simulink model "gm_Dynamic_Calculations"  (R2018a)
settings: Solver=ode3  StartTime=0.0  StopTime=0.06  RelTol=1e-3  EnableMultiTasking=on
libraries: hdlsllib x4, hdlmdlgenlib x4, simulink x1
settings Model: Creator=Estra  LastModifiedBy=Talha Rao
settings SolverCC: PositivePriorityOrder=on
settings DataIOCC: LimitDataPoints=on  SaveFormat=Array  SaveOutput=off  SaveTime=off
settings OptimizationCC: BlockReduction=off  ConditionallyExecuteInputs=off  DefaultParameterBehavior=Inlined  UseDivisionForNetSlopeComputation=on  UseFloatMulNetSlope=on  InlineInvariantSignals=on  PassReuseOutputArgsAs=Individual arguments  ExpressionDepthLimit=2147483647  ZeroExternalMemoryAtStartup=off  ZeroInternalMemoryAtStartup=off  NoFixptDivByZeroProtection=on  EfficientFloat2IntCast=on  LifeSpan=1  MaxStackSize=64
settings DebuggingCC: SignalInfNanChecking=warning  UnderspecifiedInitializationDetection=Classic  MergeDetectMultiDrivingBlocksExec=none  SolverPrmCheckMsg=warning  InheritedTsInSrcMsg=none  ParameterTunabilityLossMsg=error  UniqueDataStoreMsg=warning  AllowSymbolicDim=off  StateNameClashWarn=warning  SFUnexpectedBacktrackingDiag=warning  SFNoUnconditionalDefaultTransitionDiag=warning  SFExecutionAtInitializationDiag=none
settings HardwareCC: ProdBitPerPointer=32  ProdBitPerSizeT=32  ProdBitPerPtrDiffT=32  ProdLargestAtomicInteger=Long  ProdLargestAtomicFloat=Double  ProdWordSize=32  ProdLongLongMode=on  ProdHWDeviceType=ARM Compatible->ARM Cortex  TargetBitPerPointer=64  TargetBitPerSizeT=64  TargetBitPerPtrDiffT=64  TargetLongLongMode=on  TargetIntDivRoundTo=Zero  TargetEndianess=LittleEndian  TargetWordSize=64  TargetHWDeviceType=Custom Processor->MATLAB Host Computer  ProdEqTarget=off
settings ModelReferenceCC: PropagateSignalLabelsOutOfModel=off
settings SFSimCC: MATLABDynamicMemAlloc=off
settings RTWCC: SystemTargetFile=ert.tlc  HardwareBoard=Xilinx Zynq-7000 based board  TLCOptions="-aInlineSetEventsForThisBaseRateFcn=TLC_FALSE -aSuppressMultiTaskScheduler=TLC_FALSE  -aRateBasedStepFcn=0"  TemplateMakefile=ert_default_tmf  GenerateReport=on  Toolchain=Xilinx Software Development Kit (SDK)  IncludeHyperlinkInReport=on  LaunchReport=on  GenerateTraceInfo=on  GenerateTraceReport=on  GenerateTraceReportSl=on  GenerateTraceReportSf=on  GenerateTraceReportEml=on  GenerateCodeMetricsReport=on
settings CodeAppCC: ForceParamTrailComments=on  IgnoreCustomStorageClasses=off  OperatorAnnotations=on  SimulinkDataObjDesc=on  SFDataObjDesc=on  CustomSymbolStrGlobalVar=rt$N$M  CustomSymbolStrType=$N$M  CustomSymbolStrFcn=$N$M$F  CustomSymbolStrMacro=$N$M  InsertBlockDesc=on
settings ERTTargetCC: IncludeMdlTerminateFcn=off  CombineSignalStateStructs=on  SupportAbsoluteTime=off  SupportComplex=off  SupportNonInlinedSFcns=on  SupportVariableSizeSignals=on  InlinedParameterPlacement=NonHierarchical  ERTFilePackagingFormat=CompactWithDataFile
settings ConfigComp: CovMetricSettings=dw  CovHtmlReporting=on  CovSaveCumulativeToWorkspaceVar=on  CovSaveSingleToWorkspaceVar=on  CovExternalEMLEnable=off

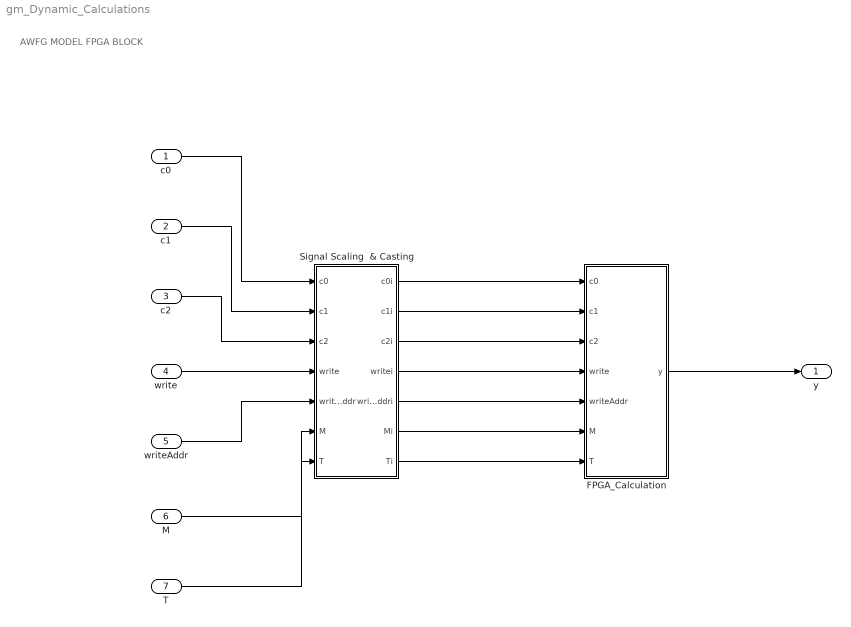
== system gm_Dynamic_Calculations ==
  note: AWFG MODEL FPGA BLOCK
  c0 : Inport  OutDataTypeStr=int32  PortDimensions=1  SampleTime=1e-08
  c1 : Inport  Port=2  OutDataTypeStr=int32  PortDimensions=1  SampleTime=1e-08
  c2 : Inport  Port=3  OutDataTypeStr=int32  PortDimensions=1  SampleTime=1e-08
  write : Inport  Port=4  OutDataTypeStr=boolean  PortDimensions=1  SampleTime=1e-08
  writeAddr : Inport  Port=5  OutDataTypeStr=uint8  PortDimensions=1  SampleTime=1e-08
  M : Inport  Port=6  OutDataTypeStr=int32  PortDimensions=1  SampleTime=1e-08
  T : Inport  Port=7  OutDataTypeStr=uint32  PortDimensions=1  SampleTime=1e-08
  FPGA_Calculation : Subsystem
  Signal Scaling  & Casting : Subsystem
  y : Outport  OutDataTypeStr=fixdt(1,27,19)  PortDimensions=[1 1]  SampleTime=[1e-08,0]
  wires:
  c0/1 -> Signal Scaling  & Casting/1(c0)
  c1/1 -> Signal Scaling  & Casting/2(c1)
  c2/1 -> Signal Scaling  & Casting/3(c2)
  write/1 -> Signal Scaling  & Casting/4(write)
  writeAddr/1 -> Signal Scaling  & Casting/5(writeAddr)
  M/1 -> Signal Scaling  & Casting/6(M)
  T/1 -> Signal Scaling  & Casting/7(T)
  FPGA_Calculation/1(y) -> y/1
  Signal Scaling  & Casting/1(c0i) -> FPGA_Calculation/1(c0)
  Signal Scaling  & Casting/2(c1i) -> FPGA_Calculation/2(c1)
  Signal Scaling  & Casting/3(c2i) -> FPGA_Calculation/3(c2)
  Signal Scaling  & Casting/4(writei) -> FPGA_Calculation/4(write)
  Signal Scaling  & Casting/5(writeAddri) -> FPGA_Calculation/5(writeAddr)
  Signal Scaling  & Casting/6(Mi) -> FPGA_Calculation/6(M)
  Signal Scaling  & Casting/7(Ti) -> FPGA_Calculation/7(T)

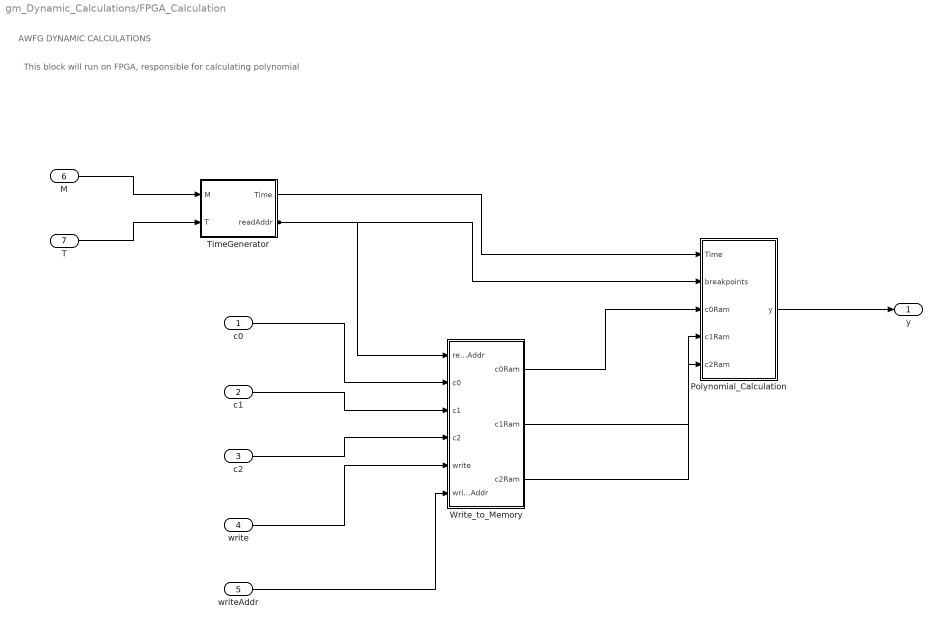
== system gm_Dynamic_Calculations/FPGA_Calculation ==
  note: AWFG DYNAMIC CALCULATIONS
  note: This block will run on FPGA, responsible for calculating polynomial
  c0 : Inport  PortDimensions=1  SampleTime=1e-08
  c1 : Inport  Port=2  PortDimensions=1  SampleTime=1e-08
  c2 : Inport  Port=3  PortDimensions=1  SampleTime=1e-08
  write : Inport  Port=4  PortDimensions=1  SampleTime=1e-08
  writeAddr : Inport  Port=5  PortDimensions=1  SampleTime=1e-08
  M : Inport  Port=6  PortDimensions=1  SampleTime=1e-08
  T : Inport  Port=7  PortDimensions=1  SampleTime=1e-08
  Polynomial_Calculation : Subsystem
  TimeGenerator : Subsystem
  Write_to_Memory : Subsystem
  y : Outport
  wires:
  c0/1 -> Write_to_Memory/2(c0)
  c1/1 -> Write_to_Memory/3(c1)
  c2/1 -> Write_to_Memory/4(c2)
  write/1 -> Write_to_Memory/5(write)
  writeAddr/1 -> Write_to_Memory/6(writeAddr)
  M/1 -> TimeGenerator/1(M)
  T/1 -> TimeGenerator/2(T)
  Polynomial_Calculation/1(y) -> y/1
  TimeGenerator/1(Time) -> Polynomial_Calculation/1(Time)
  TimeGenerator/2(readAddr) -> Polynomial_Calculation/2(breakpoints), Write_to_Memory/1(readAddr)
  Write_to_Memory/1(c0Ram) -> Polynomial_Calculation/3(c0Ram)
  Write_to_Memory/2(c1Ram) -> Polynomial_Calculation/4(c1Ram)
  Write_to_Memory/3(c2Ram) -> Polynomial_Calculation/5(c2Ram)

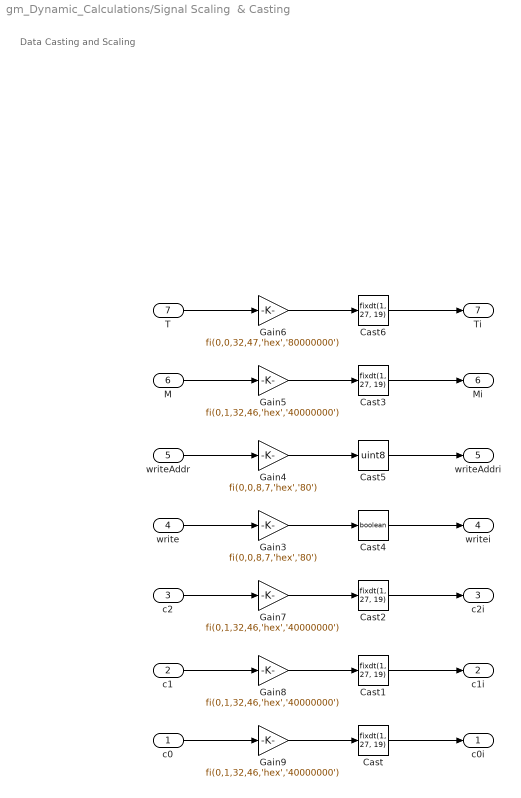
== system gm_Dynamic_Calculations/Signal Scaling  & Casting ==
  note: Data Casting and Scaling
  c0 : Inport  PortDimensions=1  SampleTime=1e-08
  c1 : Inport  Port=2  PortDimensions=1  SampleTime=1e-08
  c2 : Inport  Port=3  PortDimensions=1  SampleTime=1e-08
  write : Inport  Port=4  PortDimensions=1  SampleTime=1e-08
  writeAddr : Inport  Port=5  PortDimensions=1  SampleTime=1e-08
  M : Inport  Port=6  PortDimensions=1  SampleTime=1e-08
  T : Inport  Port=7  PortDimensions=1  SampleTime=1e-08
  Cast{,1..3,6} (5 alike) : DataTypeConversion  OutDataTypeStr=fixdt(1, 27, 19)  SampleTime=1e-08
  Cast4 : DataTypeConversion  OutDataTypeStr=boolean  SampleTime=1e-08
  Cast5 : DataTypeConversion  OutDataTypeStr=uint8  SampleTime=1e-08
  Gain3 : Gain  Gain=fi(0,0,8,7,'hex','80')  ParamDataTypeStr=fixdt(0, 8, 7)  OutDataTypeStr=fixdt(0, 8, 7)  SampleTime=1e-08
  Gain4 : Gain  Gain=fi(0,0,8,7,'hex','80')  ParamDataTypeStr=fixdt(0, 8, 7)  OutDataTypeStr=fixdt(0, 16, 7)  SampleTime=1e-08
  Gain{5,7..9} (4 alike) : Gain  Gain=fi(0,1,32,46,'hex','40000000')  ParamDataTypeStr=fixdt(1, 32, 46)  OutDataTypeStr=fixdt(1, 64, 46)  SampleTime=1e-08
  Gain6 : Gain  Gain=fi(0,0,32,47,'hex','80000000')  ParamDataTypeStr=fixdt(0, 32, 47)  OutDataTypeStr=fixdt(0, 64, 47)  SampleTime=1e-08
  c0i : Outport
  c1i : Outport  Port=2
  c2i : Outport  Port=3
  writei : Outport  Port=4
  writeAddri : Outport  Port=5
  Mi : Outport  Port=6
  Ti : Outport  Port=7
  wires:
  c0/1 -> Gain9/1
  c1/1 -> Gain8/1
  c2/1 -> Gain7/1
  write/1 -> Gain3/1
  writeAddr/1 -> Gain4/1
  M/1 -> Gain5/1
  T/1 -> Gain6/1
  Cast/1 -> c0i/1
  Cast1/1 -> c1i/1
  Cast2/1 -> c2i/1
  Cast3/1 -> Mi/1
  Cast4/1 -> writei/1
  Cast5/1 -> writeAddri/1
  Cast6/1 -> Ti/1
  Gain3/1 -> Cast4/1
  Gain4/1 -> Cast5/1
  Gain5/1 -> Cast3/1
  Gain6/1 -> Cast6/1
  Gain7/1 -> Cast2/1
  Gain8/1 -> Cast1/1
  Gain9/1 -> Cast/1

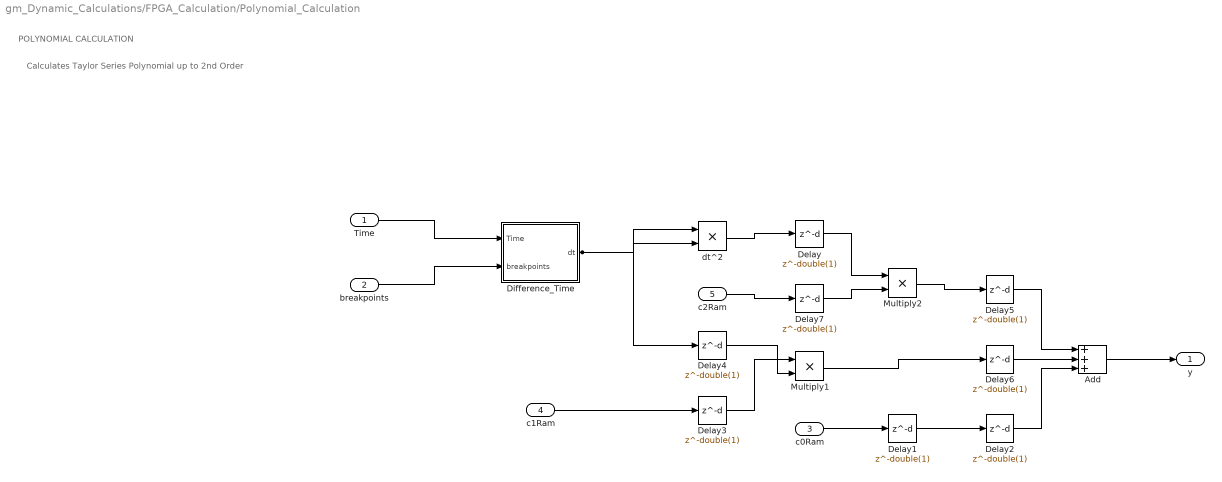
== system gm_Dynamic_Calculations/FPGA_Calculation/Polynomial_Calculation ==
  note: POLYNOMIAL CALCULATION
  note: Calculates Taylor Series Polynomial up to 2nd Order
  Time : Inport  PortDimensions=1  SampleTime=1e-08
  breakpoints : Inport  Port=2  PortDimensions=1  SampleTime=1e-08
  c0Ram : Inport  Port=3  PortDimensions=1  SampleTime=1e-08
  c1Ram : Inport  Port=4  PortDimensions=1  SampleTime=1e-08
  c2Ram : Inport  Port=5  PortDimensions=1  SampleTime=1e-08
  Add : Sum  Inputs=+++  AccumDataTypeStr=fixdt(1, 32, 19)  OutDataTypeStr=fixdt(1, 27, 19)  SampleTime=1e-08
  Delay{,1..7} (8 alike) : Delay  DelayLength=double(1)  InitialCondition=0  InputProcessing=Inherited  SampleTime=1e-08
  Difference_Time : Subsystem
  Multiply1 : Product  Inputs=**  OutDataTypeStr=fixdt(1, 27, 19)  SampleTime=1e-08
  Multiply2 : Product  Inputs=**  OutDataTypeStr=fixdt(1, 27, 19)  SampleTime=1e-08
  dt^2 : Product  Inputs=**  OutDataTypeStr=fixdt(1, 27, 19)  SampleTime=1e-08
  y : Outport
  wires:
  Time/1 -> Difference_Time/1(Time)
  breakpoints/1 -> Difference_Time/2(breakpoints)
  c0Ram/1 -> Delay1/1
  c1Ram/1 -> Delay3/1
  c2Ram/1 -> Delay7/1
  Add/1 -> y/1
  Delay/1 -> Multiply2/1
  Delay1/1 -> Delay2/1
  Delay2/1 -> Add/3
  Delay3/1 -> Multiply1/1
  Delay4/1 -> Multiply1/2
  Delay5/1 -> Add/1
  Delay6/1 -> Add/2
  Delay7/1 -> Multiply2/2
  Difference_Time/1(dt) -> dt^2/2, dt^2/1, Delay4/1
  Multiply1/1 -> Delay6/1
  Multiply2/1 -> Delay5/1
  dt^2/1 -> Delay/1

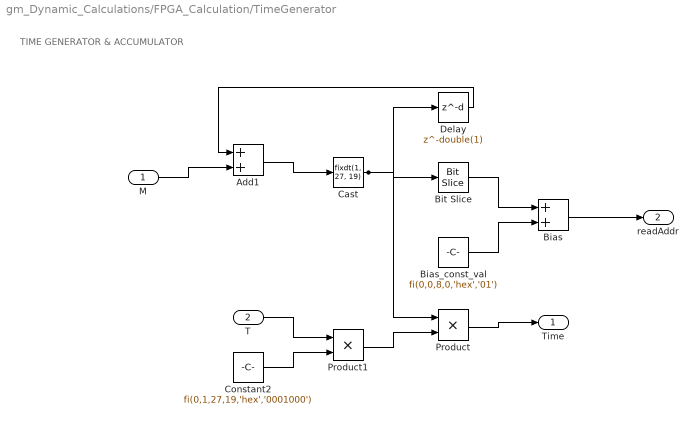
== system gm_Dynamic_Calculations/FPGA_Calculation/TimeGenerator ==
  note: TIME GENERATOR & ACCUMULATOR
  M : Inport  PortDimensions=1  SampleTime=1e-08
  T : Inport  Port=2  PortDimensions=1  SampleTime=1e-08
  Add1 : Sum  AccumDataTypeStr=fixdt(1, 32, 19)  OutDataTypeStr=fixdt(0, 26, 19)  SampleTime=1e-08
  Bias : Sum  AccumDataTypeStr=uint8  OutDataTypeStr=uint8  RndMeth=Nearest  SampleTime=1e-08
  Bias_const_val : Constant  Value=fi(0,0,8,0,'hex','01')  VectorParams1D=off  OutDataTypeStr=uint8  SampleTime=-1
  Bit Slice : hdlsllib/Logic and Bit Operations/Bit Slice  lidx=double(26)  ridx=double(19)
  Cast : DataTypeConversion  OutDataTypeStr=fixdt(1, 27, 19)  SampleTime=1e-08
  Constant2 : Constant  Value=fi(0,1,27,19,'hex','0001000')  OutDataTypeStr=fixdt(1, 27, 19)  SampleTime=-1
  Delay : Delay  DelayLength=double(1)  InitialCondition=0  InputProcessing=Inherited  SampleTime=1e-08
  Product : Product  Inputs=**  OutDataTypeStr=fixdt(1, 27, 19)  SampleTime=1e-08
  Product1 : Product  Inputs=**  OutDataTypeStr=fixdt(1, 27, 19)  SampleTime=1e-08
  Time : Outport
  readAddr : Outport  Port=2
  wires:
  M/1 -> Add1/2
  T/1 -> Product1/1
  Add1/1 -> Cast/1
  Bias/1 -> readAddr/1
  Bit Slice/1 -> Bias/1
  Cast/1 -> Product/1, Bit Slice/1, Delay/1
  Constant2/1 -> Product1/2
  Delay/1 -> Add1/1
  Product/1 -> Time/1
  Product1/1 -> Product/2
  Bias_const_val/1 -> Bias/2

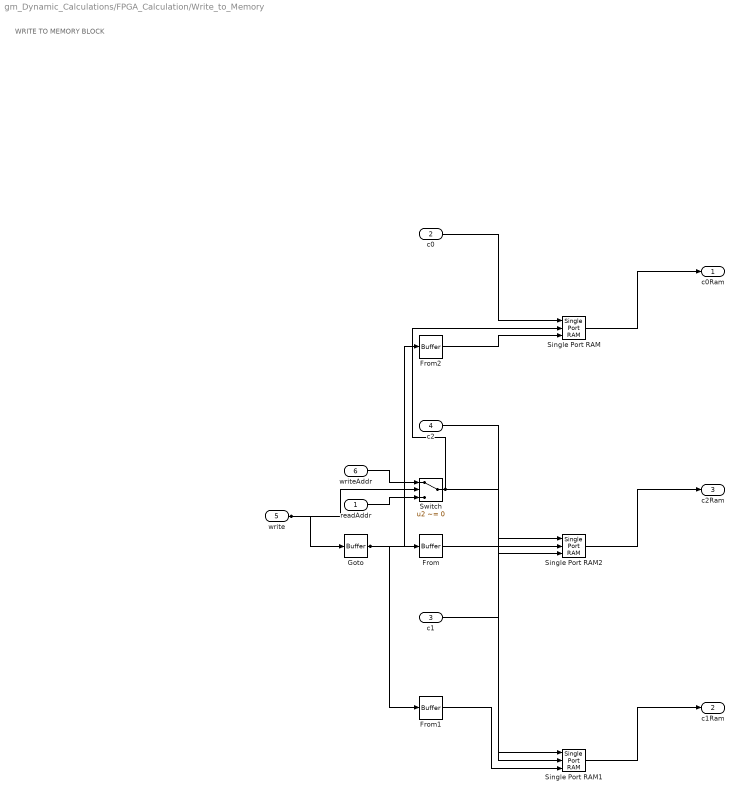
== system gm_Dynamic_Calculations/FPGA_Calculation/Write_to_Memory ==
  note: WRITE TO MEMORY BLOCK
  readAddr : Inport  PortDimensions=1  SampleTime=1e-08
  c0 : Inport  Port=2  PortDimensions=1  SampleTime=1e-08
  c1 : Inport  Port=3  PortDimensions=1  SampleTime=1e-08
  c2 : Inport  Port=4  PortDimensions=1  SampleTime=1e-08
  write : Inport  Port=5  PortDimensions=1  SampleTime=1e-08
  writeAddr : Inport  Port=6  PortDimensions=1  SampleTime=1e-08
  From : hdlmdlgenlib/Buffer
      settings: SourceProductName=HDL Coder  SourceProductBaseCode=HD
  From1 : hdlmdlgenlib/Buffer
      settings: SourceProductName=HDL Coder  SourceProductBaseCode=HD
  From2 : hdlmdlgenlib/Buffer
      settings: SourceProductName=HDL Coder  SourceProductBaseCode=HD
  Goto : hdlmdlgenlib/Buffer
      settings: SourceProductName=HDL Coder  SourceProductBaseCode=HD
  Single Port RAM : hdlsllib/HDL RAMs/Single Port RAM  ram_size=8  dout_type=New data
      settings: SourceProductName=HDL Coder  SourceProductBaseCode=HD
  Single Port RAM1 : hdlsllib/HDL RAMs/Single Port RAM  ram_size=8  dout_type=New data
      settings: SourceProductName=HDL Coder  SourceProductBaseCode=HD
  Single Port RAM2 : hdlsllib/HDL RAMs/Single Port RAM  ram_size=8  dout_type=New data
      settings: SourceProductName=HDL Coder  SourceProductBaseCode=HD
  Switch : Switch  Criteria=u2 ~= 0  Threshold=double(0)  OutDataTypeStr=uint8  SampleTime=1e-08
  c0Ram : Outport
  c1Ram : Outport  Port=2
  c2Ram : Outport  Port=3
  wires:
  readAddr/1 -> Switch/3
  c0/1 -> Single Port RAM/1
  c1/1 -> Single Port RAM1/1
  c2/1 -> Single Port RAM2/1
  write/1 -> Switch/2, Goto/1
  writeAddr/1 -> Switch/1
  From/1 -> Single Port RAM2/3
  From1/1 -> Single Port RAM1/3
  From2/1 -> Single Port RAM/3
  Single Port RAM/1 -> c0Ram/1
  Single Port RAM1/1 -> c1Ram/1
  Single Port RAM2/1 -> c2Ram/1
  Switch/1 -> Single Port RAM/2, Single Port RAM1/2, Single Port RAM2/2
  Goto/1 -> From2/1, From1/1, From/1

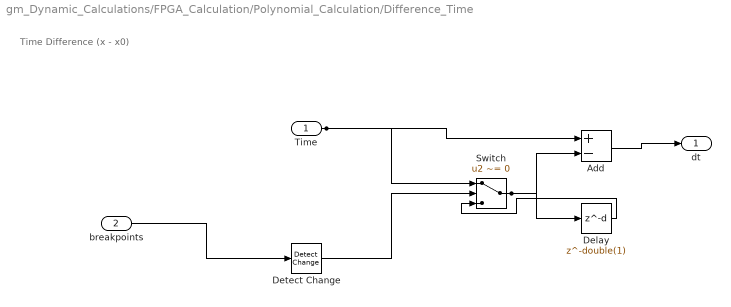
== system gm_Dynamic_Calculations/FPGA_Calculation/Polynomial_Calculation/Difference_Time ==
  note: Time Difference (x - x0)
  Time : Inport  PortDimensions=1  SampleTime=1e-08
  breakpoints : Inport  Port=2  PortDimensions=1  SampleTime=1e-08
  Add : Sum  Inputs=+-  AccumDataTypeStr=fixdt(1, 32, 19)  OutDataTypeStr=fixdt(1, 27, 19)  SampleTime=1e-08
  Delay : Delay  DelayLength=double(1)  InitialCondition=0  InputProcessing=Inherited  SampleTime=1e-08
  Detect Change : simulink/Logic and Bit Operations/Detect Change  vinit=0  OutDataTypeStr=boolean
  Switch : Switch  Criteria=u2 ~= 0  Threshold=double(0)  OutDataTypeStr=fixdt(1, 27, 19)  SampleTime=1e-08
  dt : Outport
  wires:
  Time/1 -> Switch/1, Add/1
  breakpoints/1 -> Detect Change/1
  Add/1 -> dt/1
  Delay/1 -> Switch/3
  Detect Change/1 -> Switch/2
  Switch/1 -> Add/2, Delay/1
